simulink model "Flowchart7_tmp"  (Simulink 8.3)
settings: Solver=ode45  StartTime=0.0  StopTime=10.0  RelTol=1e-3
settings Model: Creator=scaife  LastModifiedBy=bourbouh  CovSFcnEnable=on  ExtModeAutoUpdateStatusClock=off
settings DataIOCC: SignalLoggingName=sigsOut
settings OptimizationCC: InitFltsAndDblsToZero=on
settings DebuggingCC: SaveWithParameterizedLinksMsg=none  SignalResolutionControl=TryResolveAllWithWarning  SolverPrmCheckMsg=none  MultiTaskDSMMsg=warning  MultiTaskCondExecSysMsg=none  FrameProcessingCompatibilityMsg=error  StateNameClashWarn=none  StrictBusMsg=None
settings HardwareCC: TargetUnknown=on
settings SFSimCC: SimParseCustomCode=off
settings GRTTargetCC: TargetFcnLib=ansi_tfl_tmw.mat  ModelReferenceCompliant=off  GeneratePreprocessorConditionals=Use local settings  MatFileLogging=off

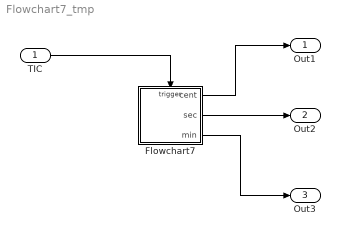
== system Flowchart7_tmp ==
  TIC : Inport
  Flowchart7 : Stateflow chart  TreatAsAtomicUnit=on
      settings: PermitHierarchicalResolution=ParametersOnly
  Out1 : Outport
  Out2 : Outport  Port=2
  Out3 : Outport  Port=3
  wires:
  TIC/1 -> Flowchart7/Trigger
  Flowchart7/1(cent) -> Out1/1
  Flowchart7/2(sec) -> Out2/1
  Flowchart7/3(min) -> Out3/1

== stateflow chart Flowchart7 ==
  (default) -> (junction 7) : TIC{cent++}
  (junction 7) -> (junction 9) [order 2]
  (junction 7) -> (junction 8) [order 1] : [cent==2]{cent=0; sec++}
  (junction 8) -> (junction 9) [order 2]
  (junction 8) -> (junction 9) [order 1] : [sec==3]{sec=0; min++}
  data: cent output int32; sec output int32; min output int32
  events: TIC input EITHER_EDGE_EVENT
